simulink model "gm_sampleModel1677_2_sub"  (R2023a)
settings: Solver=VariableStepAuto  StartTime=0.0  StopTime=10.0  RelTol=1e-3
libraries: simulink x3, hdlsllib x2
settings Model: Creator=user1  LastModifiedBy=user1
settings OptimizationCC: BlockReduction=off  ConditionallyExecuteInputs=off
settings DebuggingCC: InheritedTsInSrcMsg=none

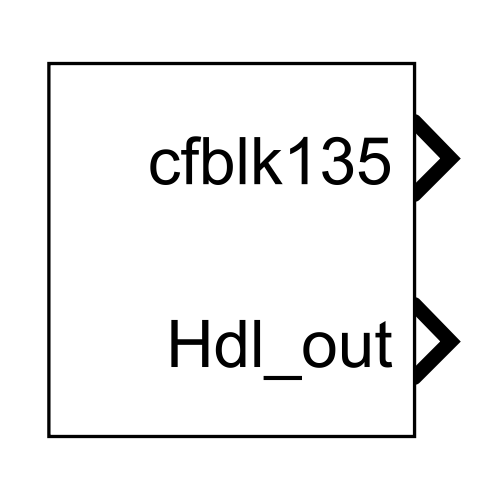
[thumbnail: Simulink's stored preview of the top-level diagram]
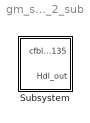
== system gm_sampleModel1677_2_sub ==
  Subsystem : Subsystem

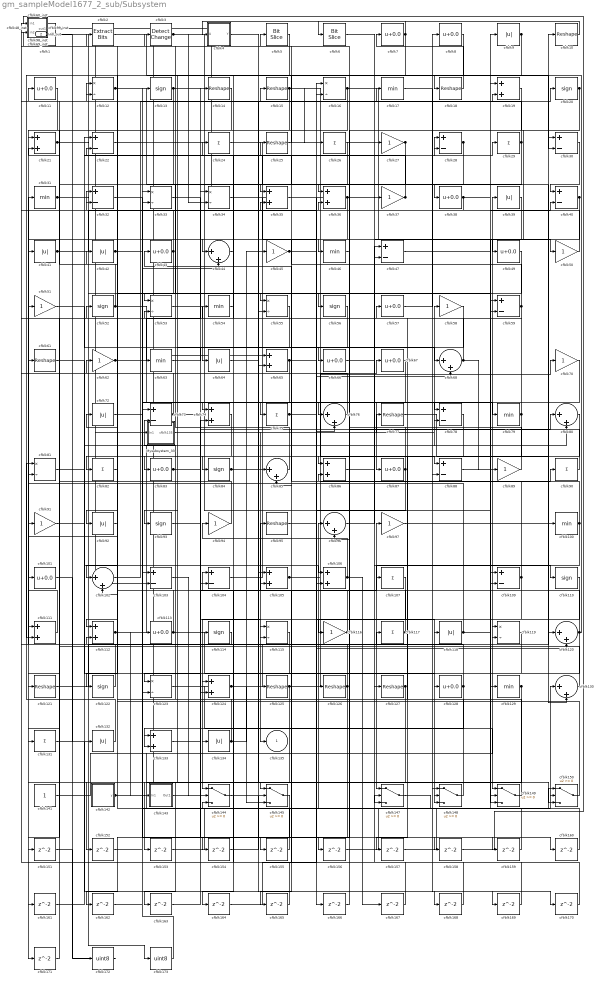
== system gm_sampleModel1677_2_sub/Subsystem ==
  Mysubsystem_33 : Subsystem
  cfblk1 : simulink/Logic and Bit Operations/Bit Set  iBit=0
      settings: LibrarySourceBlock=|
      | hdlsllib/Logic and Bit
      | Operations/Bit Set
  cfblk{10,14..15,18,25,61,77,95,121,125..127} (12 alike) : Reshape
  cfblk{17,31,46,54,63,79,100,129} (8 alike) : MinMax  OutDataTypeStr=uint8
  cfblk{7..8,11,38,43,49,57,66..67,83,87,101,113,128} (14 alike) : Bias  Bias=0.0  SaturateOnIntegerOverflow=off
  cfblk{44,68,76,80,85,96,102,120,130} (9 alike) : Sum  Inputs=|++  OutDataTypeStr=uint8
  cfblk{22,28,30,32,40,47,59,73,78,88,103..104,109} (13 alike) : Sum  Inputs=+-  OutDataTypeStr=uint8
  cfblk{19,21,35..36,65,74,86,105..106,111..112,124,133} (13 alike) : Sum  OutDataTypeStr=uint8
  cfblk{24,26,29,75,82,90,107,117,131} (9 alike) : Sum  Inputs=+  OutDataTypeStr=uint8
  cfblk{13,20,52,56,84,93,110,114,122} (9 alike) : Signum
  cfblk{12,16,33..34,53,55,81,115,119,123} (10 alike) : Product  Inputs=*/  OutDataTypeStr=uint8  RndMeth=Zero  SaturateOnIntegerOverflow=on
  cfblk{27,37,45,50..51,58,62,70,89,91,94,97,116} (13 alike) : Gain  OutDataTypeStr=uint8
  cfblk{9,39,41..42,64,72,92,118,132,134} (10 alike) : Abs  OutDataTypeStr=uint8  SaturateOnIntegerOverflow=off
  cfblk141 : Constant  OutDataTypeStr=uint8  SampleTime=-1
  cfblk142 : Subsystem  mask(Counter Free-Running){NumBits=double(16), tsamp=double(-1)}
      mask prompts: NumBits "Simulink:masks:NumberOfBits_MP"; tsamp "Simulink:masks:SampleTime_MP"
      mask help: Simulink:masks:CounterFreeRunning_MD
  cfblk143 : Subsystem
  cfblk{144..145,147..150} (6 alike) : Switch  OutDataTypeStr=uint8  SaturateOnIntegerOverflow=off  InputSameDT=off
  cfblk{151..171} (21 alike) : Delay  SampleTime=1
  cfblk172 : DataTypeConversion  OutDataTypeStr=uint8  SaturateOnIntegerOverflow=off  RndMeth=Floor
  cfblk173 : DataTypeConversion  OutDataTypeStr=uint8  SaturateOnIntegerOverflow=off  RndMeth=Floor
  cfblk2 : simulink/Logic and Bit Operations/Extract Bits  bitsToExtract=Upper half  numBits=8  bitIdxRange=[0 7]  outScalingMode=Preserve fixed-point scaling
      settings: LibrarySourceBlock=|
      | hdlsllib/Logic and Bit
      | Operations/Extract Bits
  cfblk3 : simulink/Logic and Bit Operations/Detect Change  vinit=0  OutDataTypeStr=uint8
      settings: LibrarySourceBlock=|
      | hdlsllib/Logic and Bit
      | Operations/Detect
      | Change
  cfblk4 : Subsystem  mask(Detect Fall Negative){vinit=double(0), InputProcessing=Elements as channels (sample based), OutDataTypeStr=uint8}
      mask prompts: vinit "Simulink:masks:InitialCondition_MP"; InputProcessing "Simulink:masks:InputProcessing_MP"; OutDataTypeStr "Simulink:masks:OutputDataType_MP"
      mask help: Simulink:masks:DetectFallNegative_MD
      mask init:
      | InputProcessing = 'Elements as channels (sample based)';
      | OutDataTypeStr = 'uint8';
      | vinit = double(0);
      mask TypeOptions InputProcessing: Simulink:masks:ColumnsAsChannelsFrameBased | Simulink:masks:ElementsAsChannelsSampleBased
      mask TypeOptions OutDataTypeStr: Simulink:masks:uint8 | Simulink:masks:boolean
      mask Display: fprintf('U < 0\n&  NOT\nU/z < 0')
  cfblk48_inst : Subsystem
  cfblk5 : hdlsllib/Logic and Bit Operations/Bit Slice  lidx=7  ridx=0
  cfblk6 : hdlsllib/Logic and Bit Operations/Bit Slice  lidx=7  ridx=0
  cfblk60_inst : Subsystem
  cfblk69_inst : Subsystem
  cfblk98_inst : Subsystem
  cfblk99_inst : Subsystem
  cfblk135 : Outport  OutDataTypeStr=uint8  SampleTime=1  VectorParamsAs1DForOutWhenUnconnected=off
  Hdl_out : Outport  Port=2  OutDataTypeStr=uint8  SampleTime=1
  wires:
  Mysubsystem_33/1(cfblk135) -> cfblk135/1
  cfblk1/1 -> cfblk173/1
  cfblk10/1 -> cfblk6/1
  cfblk100/1 -> cfblk43/1, cfblk147/1
  cfblk101/1 -> cfblk132/1
  cfblk102/1 -> cfblk15/1
  cfblk103/1 -> cfblk144/2
  cfblk104/1 -> cfblk29/1
  cfblk105/1 -> cfblk67/1, cfblk70/1
  cfblk106/1 -> cfblk94/1, cfblk167/1
  cfblk107/1 -> cfblk115/2
  cfblk109/1 -> cfblk86/2, cfblk148/3
  cfblk11/1 -> cfblk171/1
  cfblk110/1 -> cfblk144/1
  cfblk111/1 -> cfblk31/1
  cfblk112/1 -> cfblk30/1, cfblk58/1
  cfblk113/1 -> cfblk128/1, cfblk33/2
  cfblk114/1 -> cfblk112/2
  cfblk115/1 -> cfblk123/1
  cfblk116/1 -> cfblk95/1, cfblk72/1
  cfblk117/1 -> cfblk99_inst/2(in2), cfblk91/1
  cfblk118/1 -> cfblk19/1, cfblk81/2
  cfblk119/1 -> cfblk134/1
  cfblk12/1 -> cfblk127/1, cfblk100/1
  cfblk120/1 -> cfblk18/1, cfblk147/3, cfblk97/1
  cfblk121/1 -> cfblk117/1
  cfblk122/1 -> cfblk98_inst/2(in2)
  cfblk123/1 -> cfblk149/1
  cfblk124/1 -> cfblk39/1, cfblk145/3, cfblk10/1
  cfblk125/1 -> cfblk47/1, cfblk161/1
  cfblk126/1 -> cfblk52/1, cfblk155/1
  cfblk127/1 -> cfblk153/1, cfblk152/1
  cfblk128/1 -> cfblk133/2, cfblk101/1
  cfblk129/1 -> cfblk145/1, cfblk163/1
  cfblk13/1 -> cfblk19/2, cfblk149/3, cfblk102/2
  cfblk130/1 -> cfblk61/1
  cfblk131/1 -> cfblk168/1
  cfblk132/1 -> cfblk81/1
  cfblk133/1 -> cfblk80/1
  cfblk134/1 -> cfblk32/1, cfblk45/1
  cfblk14/1 -> cfblk151/1
  cfblk141/1 -> cfblk119/1
  cfblk142/1(y) -> cfblk148/2, cfblk144/3, cfblk113/1, cfblk119/2
  cfblk143/1(Out1) -> cfblk107/1
  cfblk144/1 -> cfblk169/1
  cfblk145/1 -> cfblk162/1
  cfblk147/1 -> cfblk130/1
  cfblk148/1 -> cfblk57/1
  cfblk149/1 -> cfblk73/2
  cfblk15/1 -> cfblk148/1, cfblk114/1, cfblk26/1
  cfblk150/1 -> cfblk62/1
  cfblk151/1 -> cfblk172/1
  cfblk152/1 -> cfblk150/2
  cfblk153/1 -> cfblk55/2
  cfblk154/1 -> cfblk150/1
  cfblk155/1 -> cfblk12/1
  cfblk156/1 -> cfblk109/2
  cfblk157/1 -> cfblk59/1
  cfblk158/1 -> cfblk69_inst/1(in1)
  cfblk159/1 -> cfblk96/1
  cfblk16/1 -> cfblk21/1, cfblk109/1
  cfblk160/1 -> cfblk73/1
  cfblk161/1 -> cfblk28/1
  cfblk162/1 -> cfblk44/2
  cfblk163/1 -> cfblk74/2
  cfblk164/1 -> cfblk16/2
  cfblk165/1 -> cfblk104/1
  cfblk166/1 -> cfblk36/2
  cfblk167/1 -> cfblk105/2
  cfblk168/1 -> cfblk147/2
  cfblk169/1 -> cfblk98_inst/1(in1)
  cfblk17/1 -> cfblk170/1
  cfblk170/1 -> cfblk48_inst/1(in1)
  cfblk171/1 -> cfblk111/1
  cfblk172/1 -> cfblk1/1
  cfblk173/1 -> cfblk13/1
  cfblk18/1 -> cfblk7/1
  cfblk19/1 -> cfblk36/1
  cfblk2/1 -> cfblk30/2
  cfblk20/1 -> cfblk49/1, cfblk116/1
  cfblk21/1 -> cfblk28/2, cfblk121/1
  cfblk22/1 -> cfblk105/1
  cfblk24/1 -> cfblk38/1
  cfblk25/1 -> cfblk5/1
  cfblk26/1 -> cfblk41/1
  cfblk27/1 -> cfblk84/1, cfblk122/1
  cfblk28/1 -> cfblk53/1, cfblk164/1
  cfblk29/1 -> cfblk69_inst/2(in2), cfblk56/1
  cfblk3/1 -> cfblk55/1, cfblk34/2
  cfblk30/1 -> cfblk40/1
  cfblk31/1 -> cfblk65/2, cfblk59/2
  cfblk32/1 -> cfblk76/1
  cfblk33/1 -> cfblk115/1
  cfblk34/1 -> cfblk166/1
  cfblk35/1 -> cfblk120/2
  cfblk36/1 -> cfblk47/2, cfblk46/1
  cfblk37/1 -> cfblk22/2, cfblk3/1
  cfblk38/1 -> cfblk9/1, cfblk35/2
  cfblk39/1 -> cfblk75/1
  cfblk4/1(Y) -> cfblk150/3
  cfblk40/1 -> cfblk86/1, cfblk131/1
  cfblk41/1 -> cfblk88/2, cfblk16/1
  cfblk42/1 -> cfblk76/2, cfblk160/1
  cfblk43/1 -> cfblk11/1, cfblk103/1
  cfblk44/1 -> cfblk124/1
  cfblk45/1 -> cfblk85/2, cfblk118/1
  cfblk46/1 -> cfblk96/2
  cfblk47/1 -> cfblk129/1
  cfblk48_inst/1(out1) -> cfblk145/2, cfblk103/2, cfblk37/1
  cfblk49/1 -> cfblk112/1
  cfblk5/1 -> cfblk44/1
  cfblk50/1 -> cfblk48_inst/2(in2)
  cfblk51/1 -> cfblk66/1
  cfblk52/1 -> cfblk85/1, cfblk78/1, cfblk21/2
  cfblk53/1 -> cfblk64/1
  cfblk54/1 -> cfblk74/1
  cfblk55/1 -> cfblk83/1
  cfblk56/1 -> cfblk154/1
  cfblk57/1 -> cfblk8/1
  cfblk58/1 -> cfblk133/1
  cfblk59/1 -> cfblk25/1, cfblk53/2
  cfblk6/1 -> cfblk50/1
  cfblk60_inst/1(out1) -> cfblk125/1, Hdl_out/1
  cfblk61/1 -> cfblk104/2
  cfblk62/1 -> cfblk14/1, cfblk12/2
  cfblk63/1 -> cfblk68/1
  cfblk64/1 -> cfblk149/2
  cfblk65/1 -> cfblk126/1, cfblk123/2
  cfblk66/1 -> cfblk88/1
  cfblk67/1 -> cfblk165/1
  cfblk68/1 -> cfblk99_inst/1(in1), cfblk89/1, cfblk24/1
  cfblk69_inst/1(out1) -> cfblk27/1
  cfblk7/1 -> cfblk4/1(U), cfblk82/1
  cfblk70/1 -> cfblk87/1
  cfblk72/1 -> cfblk63/1
  cfblk73/1 -> cfblk93/1, cfblk42/1, cfblk158/1
  cfblk74/1 -> cfblk102/1
  cfblk75/1 -> cfblk20/1, cfblk79/1
  cfblk76/1 -> cfblk60_inst/2(in2)
  cfblk77/1 -> cfblk120/1
  cfblk78/1 -> cfblk156/1
  cfblk79/1 -> cfblk92/1, cfblk33/1
  cfblk8/1 -> cfblk111/2
  cfblk80/1 -> cfblk157/1
  cfblk81/1 -> cfblk124/2
  cfblk82/1 -> cfblk32/2
  cfblk83/1 -> cfblk77/1, cfblk106/1
  cfblk84/1 -> cfblk78/2, cfblk17/1
  cfblk85/1 -> cfblk22/1
  cfblk86/1 -> cfblk110/1
  cfblk87/1 -> cfblk106/2, cfblk34/1
  cfblk88/1 -> cfblk40/2
  cfblk89/1 -> cfblk60_inst/1(in1)
  cfblk9/1 -> cfblk35/1, cfblk143/1(In1)
  cfblk90/1 -> cfblk54/1
  cfblk91/1 -> cfblk80/2
  cfblk92/1 -> cfblk2/1
  cfblk93/1 -> cfblk159/1
  cfblk94/1 -> cfblk51/1
  cfblk95/1 -> cfblk68/2
  cfblk96/1 -> cfblk90/1
  cfblk97/1 -> cfblk130/2
  cfblk98_inst/1(out1) -> cfblk65/1
  cfblk99_inst/1(out1) -> Mysubsystem_33/1(In1)

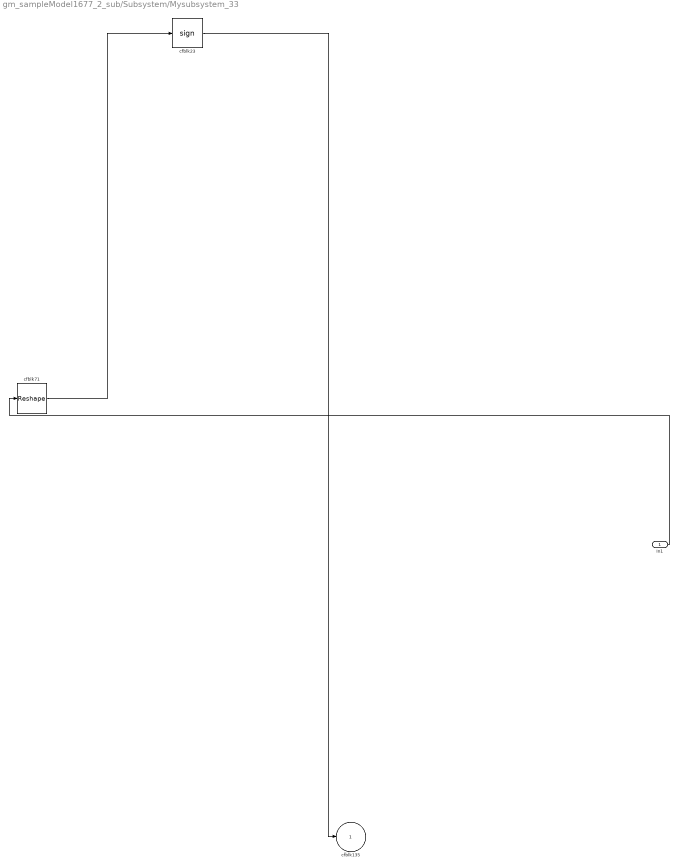
== system gm_sampleModel1677_2_sub/Subsystem/Mysubsystem_33 ==
  In1 : Inport  OutDataTypeStr=uint8  PortDimensions=1  SampleTime=1
  cfblk23 : Signum
  cfblk71 : Reshape
  cfblk135 : Outport  SampleTime=1  VectorParamsAs1DForOutWhenUnconnected=off
  wires:
  In1/1 -> cfblk71/1
  cfblk23/1 -> cfblk135/1
  cfblk71/1 -> cfblk23/1

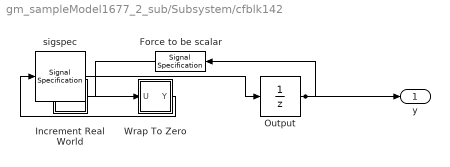
== system gm_sampleModel1677_2_sub/Subsystem/cfblk142 ==
  Force to be scalar : SignalSpecification  DisableCoverage=on  Dimensions=1
  Increment Real World : Subsystem  mask(Real World Value Increment){}
      mask help: Simulink:masks:RealWorldValueIncrement_MD
      mask Display: disp('V++')
  Output : UnitDelay  InitialCondition=0.0  SampleTime=tsamp  HasFrameUpgradeWarning=on
  Wrap To Zero : Subsystem  mask(Wrap To Zero){Threshold=double(65535)}
      mask prompts: Threshold "Simulink:masks:Threshold_MP"
      mask help: Simulink:masks:WrapToZero_MD
  sigspec : SignalSpecification  OutDataTypeStr=uint16  Dimensions=1
  y : Outport  SampleTime=1
  wires:
  Force to be scalar/1 -> Increment Real World/1(u)
  Increment Real World/1(y) -> Wrap To Zero/1(U)
  Output/1 -> Force to be scalar/1, y/1
  Wrap To Zero/1(Y) -> sigspec/1
  sigspec/1 -> Output/1

== system gm_sampleModel1677_2_sub/Subsystem/cfblk143 ==
  In1 : Inport  OutDataTypeStr=uint8  PortDimensions=1  SampleTime=1
  Out1 : Outport  SampleTime=1
  wires:
  In1/1 -> Out1/1

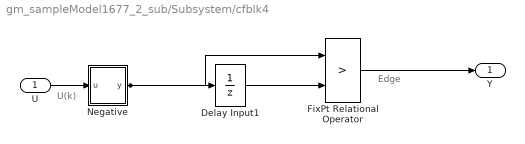
== system gm_sampleModel1677_2_sub/Subsystem/cfblk4 ==
  note: U(k)
  note: Edge
  U : Inport  OutDataTypeStr=uint8  SampleTime=1
  Delay Input1 : UnitDelay  Description=Store in Global RAM  DisableCoverage=on  InitialCondition=vinit  SampleTime=-1  HasFrameUpgradeWarning=on
  FixPt Relational Operator : RelationalOperator  Operator=>  OutDataTypeStr=fixdt(0, 8)  ZeroCross=off  InputSameDT=off
  Negative : Subsystem  mask(Compare To Zero){relop=<, OutDataTypeStr=boolean, ZeroCross=off}
      mask prompts: relop "Simulink:masks:Operator_MP"; OutDataTypeStr "Simulink:masks:OutputDataType_MP"; ZeroCross "Simulink:masks:EnableZerocrossingDetection_MP"
      mask help: Simulink:masks:CompareToZero_MD
      mask init:
      | OutDataTypeStr = 'boolean';
      | ZeroCross = 'off';
      | blkName = 'sampleModel1677_2_sub/Subsystem/cfblk4/Negative';
      | relop = '<';
      | setValue = 'boolean';
      mask TypeOptions relop: == | ~= | < | <= | >= | >
      mask TypeOptions OutDataTypeStr: Simulink:masks:uint8 | Simulink:masks:boolean
      mask Callback ZeroCross: sl('zeroCrossEnable', gcbh);
      mask Display: disp([relop,' 0'])
  Y : Outport  SampleTime=1
  wires:
  U/1 -> Negative/1(u)
  Delay Input1/1 -> FixPt Relational Operator/2
  FixPt Relational Operator/1 -> Y/1
  Negative/1(y) -> FixPt Relational Operator/1, Delay Input1/1

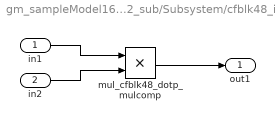
== system gm_sampleModel1677_2_sub/Subsystem/cfblk48_inst ==
  in1 : Inport  OutDataTypeStr=uint8  SampleTime=1
  in2 : Inport  Port=2  OutDataTypeStr=uint8  SampleTime=1
  mul_cfblk48_dotp_mulcomp : Product  Inputs=**  OutDataTypeStr=uint8  SampleTime=1
  out1 : Outport  OutDataTypeStr=uint8  SampleTime=1
  wires:
  in1/1 -> mul_cfblk48_dotp_mulcomp/1
  in2/1 -> mul_cfblk48_dotp_mulcomp/2
  mul_cfblk48_dotp_mulcomp/1 -> out1/1

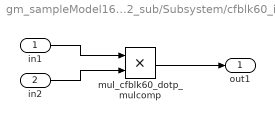
== system gm_sampleModel1677_2_sub/Subsystem/cfblk60_inst ==
  in1 : Inport  OutDataTypeStr=uint8  SampleTime=1
  in2 : Inport  Port=2  OutDataTypeStr=uint8  SampleTime=1
  mul_cfblk60_dotp_mulcomp : Product  Inputs=**  OutDataTypeStr=uint8  SampleTime=1
  out1 : Outport  OutDataTypeStr=uint8  SampleTime=1
  wires:
  in1/1 -> mul_cfblk60_dotp_mulcomp/1
  in2/1 -> mul_cfblk60_dotp_mulcomp/2
  mul_cfblk60_dotp_mulcomp/1 -> out1/1

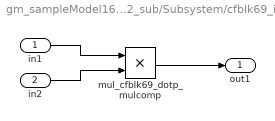
== system gm_sampleModel1677_2_sub/Subsystem/cfblk69_inst ==
  in1 : Inport  OutDataTypeStr=uint8  SampleTime=1
  in2 : Inport  Port=2  OutDataTypeStr=uint8  SampleTime=1
  mul_cfblk69_dotp_mulcomp : Product  Inputs=**  OutDataTypeStr=uint8  SampleTime=1
  out1 : Outport  OutDataTypeStr=uint8  SampleTime=1
  wires:
  in1/1 -> mul_cfblk69_dotp_mulcomp/1
  in2/1 -> mul_cfblk69_dotp_mulcomp/2
  mul_cfblk69_dotp_mulcomp/1 -> out1/1

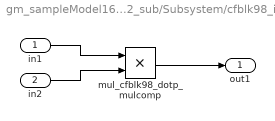
== system gm_sampleModel1677_2_sub/Subsystem/cfblk98_inst ==
  in1 : Inport  OutDataTypeStr=uint8  SampleTime=1
  in2 : Inport  Port=2  OutDataTypeStr=uint8  SampleTime=1
  mul_cfblk98_dotp_mulcomp : Product  Inputs=**  OutDataTypeStr=uint8  SampleTime=1
  out1 : Outport  OutDataTypeStr=uint8  SampleTime=1
  wires:
  in1/1 -> mul_cfblk98_dotp_mulcomp/1
  in2/1 -> mul_cfblk98_dotp_mulcomp/2
  mul_cfblk98_dotp_mulcomp/1 -> out1/1

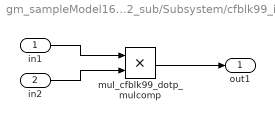
== system gm_sampleModel1677_2_sub/Subsystem/cfblk99_inst ==
  in1 : Inport  OutDataTypeStr=uint8  SampleTime=1
  in2 : Inport  Port=2  OutDataTypeStr=uint8  SampleTime=1
  mul_cfblk99_dotp_mulcomp : Product  Inputs=**  OutDataTypeStr=uint8  SampleTime=1
  out1 : Outport  OutDataTypeStr=uint8  SampleTime=1
  wires:
  in1/1 -> mul_cfblk99_dotp_mulcomp/1
  in2/1 -> mul_cfblk99_dotp_mulcomp/2
  mul_cfblk99_dotp_mulcomp/1 -> out1/1

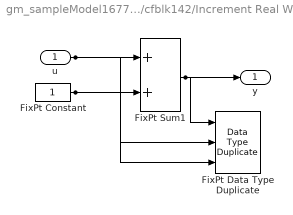
== system gm_sampleModel1677_2_sub/Subsystem/cfblk142/Increment Real World ==
  u : Inport  OutDataTypeStr=uint16  SampleTime=1
  FixPt Constant : Constant  DisableCoverage=on  OutDataTypeStr=Inherit: Inherit via back propagation  SampleTime=-1
  FixPt Data Type Duplicate : DataTypeDuplicate  DisableCoverage=on  NumInputPorts=3
  FixPt Sum1 : Sum  InputSameDT=on  OutDataTypeStr=Inherit: Inherit via back propagation  LockScale=on
  y : Outport  SampleTime=1
  wires:
  u/1 -> FixPt Sum1/1, FixPt Data Type Duplicate/2
  FixPt Constant/1 -> FixPt Sum1/2, FixPt Data Type Duplicate/3
  FixPt Sum1/1 -> FixPt Data Type Duplicate/1, y/1

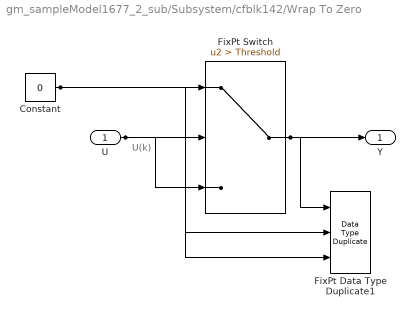
== system gm_sampleModel1677_2_sub/Subsystem/cfblk142/Wrap To Zero ==
  note: U(k)
  U : Inport  OutDataTypeStr=uint16  SampleTime=1
  Constant : Constant  DisableCoverage=on  Value=0  OutDataTypeStr=Inherit: Inherit via back propagation  SampleTime=-1
  FixPt Data Type Duplicate1 : DataTypeDuplicate  DisableCoverage=on  NumInputPorts=3
  FixPt Switch : Switch  Criteria=u2 > Threshold  Threshold=Threshold  OutDataTypeStr=Inherit: Inherit via back propagation  ZeroCross=off  SaturateOnIntegerOverflow=off  InputSameDT=off
  Y : Outport  SampleTime=1
  wires:
  U/1 -> FixPt Switch/3, FixPt Switch/2, FixPt Data Type Duplicate1/2
  Constant/1 -> FixPt Switch/1, FixPt Data Type Duplicate1/3
  FixPt Switch/1 -> FixPt Data Type Duplicate1/1, Y/1

== system gm_sampleModel1677_2_sub/Subsystem/cfblk4/Negative ==
  u : Inport  OutDataTypeStr=uint8  SampleTime=1
  Compare : RelationalOperator  Operator=<  OutDataTypeStr=boolean  ZeroCross=off
  Constant : Constant  DisableCoverage=on  Value=0  OutDataTypeStr=Inherit: Inherit via back propagation  SampleTime=-1  PreserveConstantTs=on
  y : Outport  SampleTime=1
  wires:
  u/1 -> Compare/1
  Compare/1 -> y/1
  Constant/1 -> Compare/2
